simulink model "flyball"  (R2024b)
settings: Solver=ode4  StartTime=0.0  StopTime=10.0  FixedStep=sample_t  RelTol=1e-3
values from neighbouring files (symbols this model uses):
  control = 0    [init.m]
  g = -9.8    [init.m]
  target_t = 7    [init.m]
  target_vy = -30    [init.m]
  target_y = 0    [init.m]
  vy0 = 0    [init.m]
  y0 = 100    [init.m]
libraries: simulink x2
settings Model: DataDictionary=flyballDB.sldd  TunableVars=control,target_t,target_vy,target_y  TunableVarsStorageClass=Auto,Auto,Auto,Auto  TunableVarsTypeQualifier=,,,  Creator=dell  LastModifiedBy=dell
settings OptimizationCC: DefaultParameterBehavior=Inlined  EnhancedBackFolding=on  PassReuseOutputArgsAs=Individual arguments  ZeroExternalMemoryAtStartup=off  ZeroInternalMemoryAtStartup=off  InitFltsAndDblsToZero=on  OptimizeBlockOrder=speed  DifferentSizesBufferReuse=on  OptimizationCustomize=off  EfficientTunableParamExpr=on
settings DebuggingCC: ParameterTunabilityLossMsg=error
settings HardwareCC: ProdLongLongMode=on  TargetLongLongMode=on
settings SFSimCC: MATLABDynamicMemAlloc=off
settings RTWCC: Description=Embedded Coder  SystemTargetFile=ert.tlc  GenCodeOnly=on  PackageGeneratedCodeAndArtifacts=on  TemplateMakefile=ert_default_tmf  Toolchain=Microsoft Visual Studio Project 2019 | CMake (64-bit Windows)  BuildConfiguration=Release  TargetLang=C++
settings CodeAppCC: GenerateComments=off  IgnoreCustomStorageClasses=off  OperatorAnnotations=on  SimulinkDataObjDesc=on  SFDataObjDesc=on  SimulinkBlockComments=off
settings ERTTargetCC: TargetLangStandard=C++11 (ISO)  GenerateSampleERTMain=on  CodeInterfacePackaging=C++ class  SupportComplex=off  SupportContinuousTime=on  RootIOFormat=Structure reference  ERTCustomFileTemplate=example_file_process.tlc

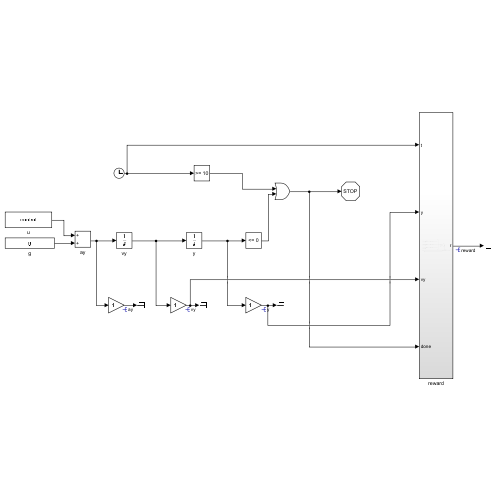
[thumbnail: Simulink's stored preview of the top-level diagram]
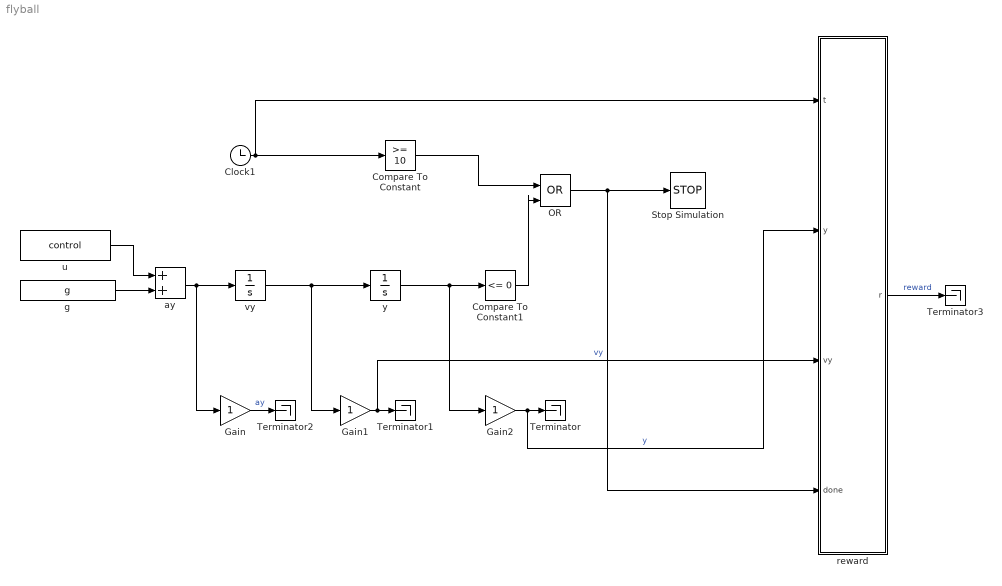
== system flyball ==
  Clock1 : Clock
  Compare To Constant : simulink/Logic and Bit Operations/Compare To Constant  relop=>=  const=10  OutDataTypeStr=boolean
  Compare To Constant1 : simulink/Logic and Bit Operations/Compare To Constant  relop=<=  const=0  OutDataTypeStr=boolean
  Gain : Gain
  Gain1 : Gain
  Gain2 : Gain
  OR : Logic  Operator=OR  IconShape=distinctive  AllPortsSameDT=off  OutDataTypeStr=boolean
  Stop Simulation : Stop
  Terminator{,1..3} (4 alike) : Terminator
  ay : Sum
  g : Constant  Value=g
  reward : Subsystem
  u : Constant  Value=control
  vy : Integrator  InitialCondition=vy0
  y : Integrator  InitialCondition=y0
  wires:
  vy/1 -> Gain1/1, y/1
  g/1 -> ay/2
  u/1 -> ay/1
  y/1 -> Gain2/1, Compare To Constant1/1
  Compare To Constant/1 -> OR/1
  Compare To Constant1/1 -> OR/2
  OR/1 -> reward/4(done), Stop Simulation/1
  ay/1 -> vy/1, Gain/1
  Gain/1 -> Terminator2/1  "ay"
  Gain1/1 -> reward/3(vy), Terminator1/1  "vy"
  Gain2/1 -> reward/2(y), Terminator/1  "y"
  Clock1/1 -> reward/1(t), Compare To Constant/1
  reward/1(r) -> Terminator3/1  "reward"

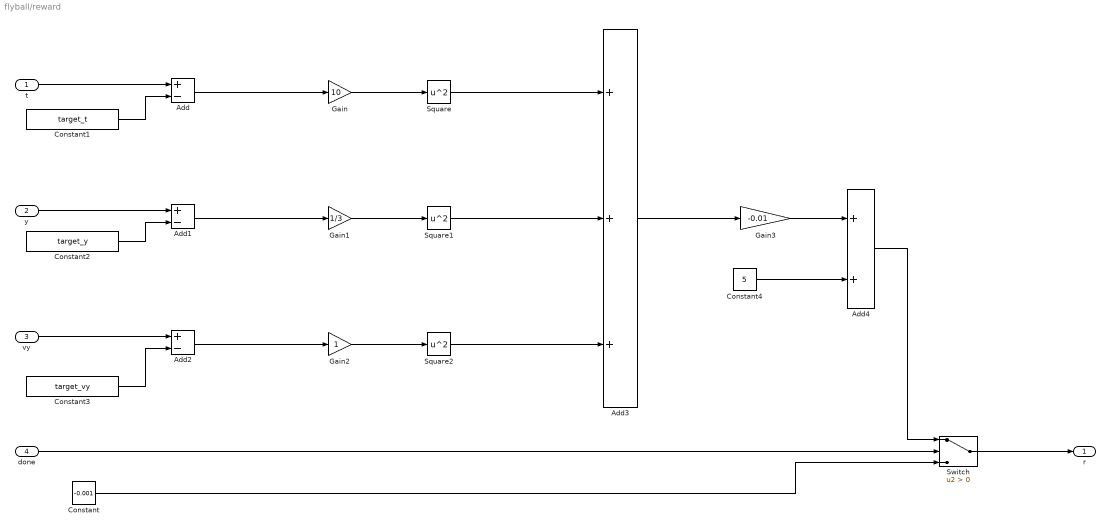
== system flyball/reward ==
  t : Inport
  y : Inport  Port=2
  vy : Inport  Port=3
  done : Inport  Port=4
  Add : Sum  Inputs=+-
  Add1 : Sum  Inputs=+-
  Add2 : Sum  Inputs=+-
  Add3 : Sum  Inputs=+++
  Add4 : Sum
  Constant : Constant  Value=-0.001
  Constant1 : Constant  Value=target_t
  Constant2 : Constant  Value=target_y
  Constant3 : Constant  Value=target_vy
  Constant4 : Constant  Value=5
  Gain : Gain  Gain=10
  Gain1 : Gain  Gain=1/3
  Gain2 : Gain
  Gain3 : Gain  Gain=-0.01
  Square : Math  Operator=square
  Square1 : Math  Operator=square
  Square2 : Math  Operator=square
  Switch : Switch  Criteria=u2 > Threshold  SaturateOnIntegerOverflow=off  InputSameDT=off
  r : Outport
  wires:
  done/1 -> Switch/2
  Constant/1 -> Switch/3
  t/1 -> Add/1
  Constant1/1 -> Add/2
  y/1 -> Add1/1
  Constant2/1 -> Add1/2
  vy/1 -> Add2/1
  Constant3/1 -> Add2/2
  Add/1 -> Gain/1
  Add1/1 -> Gain1/1
  Add2/1 -> Gain2/1
  Gain/1 -> Square/1
  Gain1/1 -> Square1/1
  Gain2/1 -> Square2/1
  Square/1 -> Add3/1
  Square2/1 -> Add3/3
  Square1/1 -> Add3/2
  Add3/1 -> Gain3/1
  Gain3/1 -> Add4/1
  Constant4/1 -> Add4/2
  Add4/1 -> Switch/1
  Switch/1 -> r/1
